simulink model "gm_flyback_pid_vnl"  (R2021b)
settings: Solver=FixedStepDiscrete  StartTime=0.0  StopTime=100e-3  RelTol=1e-3
undefined symbols (not defined in the file or in its folder): DiscIntNeverNeededParam
libraries: simulink x3
Description:
  | Symmetric FIR Filter
  | This example shows how to use HDL Coder(TM) to check, generate,
  | and verify HDL for a fixed-point symmetric FIR filter.
settings Model: Creator=The MathWorks, Inc.  LastModifiedBy=Marco Milanesi
settings SolverCC: AlgebraicLoopSolver=TrustRegion  AutoInsertRateTranBlk=on
settings DataIOCC: LimitDataPoints=on  SaveFormat=Array  SaveOutput=off  SignalLogging=off  SaveTime=off  ReturnWorkspaceOutputs=off  SignalLoggingName=logsOut
settings OptimizationCC: BlockReduction=off  BooleanDataType=off  ConditionallyExecuteInputs=off  DefaultParameterBehavior=Inlined  InheritOutputTypeSmallerThanSingle=on  InlineInvariantSignals=on  ExpressionDepthLimit=2147483647  InitFltsAndDblsToZero=on  LifeSpan=inf  BufferReusableBoundary=off
settings DebuggingCC: AlgebraicLoopMsg=error  SaveWithParameterizedLinksMsg=none  UnderspecifiedInitializationDetection=Classic  MergeDetectMultiDrivingBlocksExec=none  CheckExecutionContextPreStartOutputMsg=on  SignalResolutionControl=TryResolveAllWithWarning  InheritedTsInSrcMsg=none  MultiTaskDSMMsg=warning  MultiTaskCondExecSysMsg=none  SingleTaskRateTransMsg=error  IntegerOverflowMsg=none  ParameterPrecisionLossMsg=none  FcnCallInpInsideContextMsg=warning  BusObjectLabelMismatch=none  StateNameClashWarn=warning  SFUnexpectedBacktrackingDiag=warning  SFNoUnconditionalDefaultTransitionDiag=warning  SFExecutionAtInitializationDiag=none  SFMachineParentedDataDiag=warning  IntegerSaturationMsg=none  ArithmeticOperatorsInVariantConditions=warning
settings HardwareCC: ProdBitPerPointer=32  ProdBitPerSizeT=32  ProdBitPerPtrDiffT=32  ProdLargestAtomicFloat=None  ProdIntDivRoundTo=Undefined  ProdEndianess=Unspecified  ProdWordSize=32  ProdHWDeviceType=ASIC/FPGA  TargetUnknown=on  ProdEqTarget=off
settings ModelReferenceCC: PropagateSignalLabelsOutOfModel=off
settings SFSimCC: SimUseLocalCustomCode=off  CustomCodeUndefinedFunction=UseInterfaceOnly
settings RTWCC: RTWUseLocalCustomCode=off
settings CodeAppCC: StateflowObjectComments=on
settings GRTTargetCC: TargetFcnLib=ansi_tfl_tmw.mat  TargetLangStandard=C89/C90 (ANSI)  CombineOutputUpdateFcns=off  GRTInterface=on
settings ConfigComp: CovMetricSettings=dw  CovSaveCumulativeToWorkspaceVar=on  CovSaveSingleToWorkspaceVar=on  CovExternalEMLEnable=off

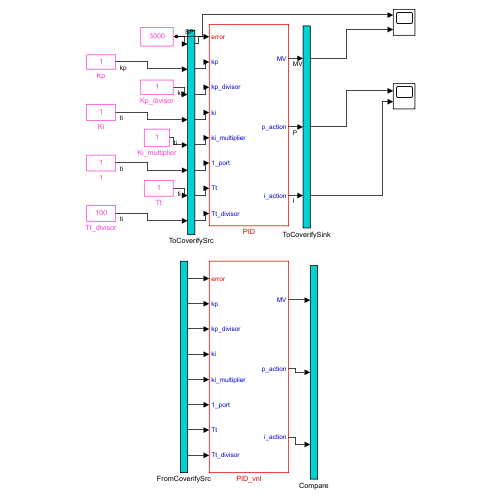
[thumbnail: Simulink's stored preview of the top-level diagram]
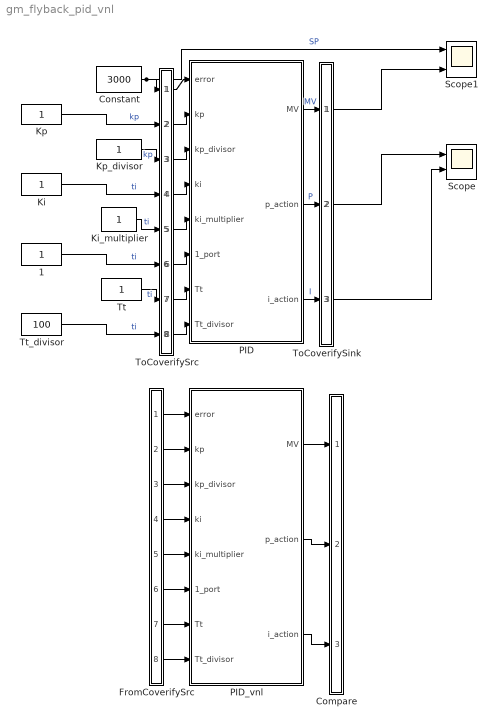
== system gm_flyback_pid_vnl ==
  1 : Constant  OutDataTypeStr=fixdt(1,16,0)
  Compare : Subsystem
      mask Display: disp('')
  Constant : Constant  Value=3000  OutDataTypeStr=fixdt(1,16,0)
  FromCoverifySrc : Subsystem
      mask Display: disp('')
  Ki : Constant  OutDataTypeStr=fixdt(1,16,0)
  Ki_multiplier : Constant  OutDataTypeStr=fixdt(1,16,0)
  Kp : Constant  OutDataTypeStr=fixdt(1,16,0)
  Kp_divisor : Constant  OutDataTypeStr=fixdt(1,16,0)
  PID : Subsystem
  PID_vnl : Subsystem
  Scope : Scope  NumInputPorts=2
  Scope1 : Scope  NumInputPorts=2
  ToCoverifySink : Subsystem
      mask Display: disp('')
  ToCoverifySrc : Subsystem
      mask Display: disp('')
  Tt : Constant  OutDataTypeStr=fixdt(1,16,0)
  Tt_divisor : Constant  Value=100  OutDataTypeStr=fixdt(1,16,0)
  wires:
  Constant/1 -> Scope1/1, ToCoverifySrc/1(in1)  "SP"
  ToCoverifySrc/1(out1) -> PID/1(error)
  ToCoverifySrc/2(out2) -> PID/2(kp)
  ToCoverifySrc/3(out3) -> PID/3(kp_divisor)
  ToCoverifySrc/4(out4) -> PID/4(ki)
  ToCoverifySrc/5(out5) -> PID/5(ki_multiplier)
  ToCoverifySrc/6(out6) -> PID/6(1_port)
  ToCoverifySrc/7(out7) -> PID/7(Tt)
  ToCoverifySrc/8(out8) -> PID/8(Tt_divisor)
  PID/1(MV) -> ToCoverifySink/1(in1)  "MV"
  PID/2(p_action) -> ToCoverifySink/2(in2)  "P"
  PID/3(i_action) -> ToCoverifySink/3(in3)  "I"
  Kp/1 -> ToCoverifySrc/2(in2)  "kp"
  Kp_divisor/1 -> ToCoverifySrc/3(in3)  "kp"
  Ki/1 -> ToCoverifySrc/4(in4)  "ti"
  Ki_multiplier/1 -> ToCoverifySrc/5(in5)  "ti"
  1/1 -> ToCoverifySrc/6(in6)  "ti"
  Tt/1 -> ToCoverifySrc/7(in7)  "ti"
  Tt_divisor/1 -> ToCoverifySrc/8(in8)  "ti"
  ToCoverifySink/1(out1) -> Scope1/2
  ToCoverifySink/2(out2) -> Scope/1
  ToCoverifySink/3(out3) -> Scope/2
  FromCoverifySrc/1(out1) -> PID_vnl/1(error)
  FromCoverifySrc/2(out2) -> PID_vnl/2(kp)
  FromCoverifySrc/3(out3) -> PID_vnl/3(kp_divisor)
  FromCoverifySrc/4(out4) -> PID_vnl/4(ki)
  FromCoverifySrc/5(out5) -> PID_vnl/5(ki_multiplier)
  FromCoverifySrc/6(out6) -> PID_vnl/6(1_port)
  FromCoverifySrc/7(out7) -> PID_vnl/7(Tt)
  FromCoverifySrc/8(out8) -> PID_vnl/8(Tt_divisor)
  PID_vnl/1(MV) -> Compare/1(in1)
  PID_vnl/2(p_action) -> Compare/2(in2)
  PID_vnl/3(i_action) -> Compare/3(in3)

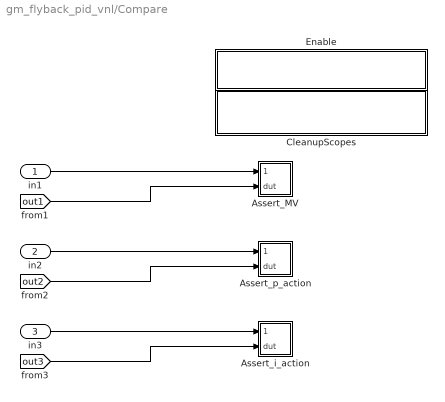
== system gm_flyback_pid_vnl/Compare ==
  in1 : Inport
  in2 : Inport  Port=2
  in3 : Inport  Port=3
  Assert_MV : Subsystem
  Assert_i_action : Subsystem
  Assert_p_action : Subsystem
  CleanupScopes : Subsystem
      settings: OpenFcn=|
      | blkName = gcb; %self block
      | idx = regexp(blkName, '/CleanupScopes$', 'once');
      | blkParent = blkName(1:idx-1);
      | blks=find_system(blkParent, 'LookUnderMasks', 'all','blocktype', 'Scope');
      | for itr = 1:length(blks)
      | 	 hScopeCfg = get_param(blks{itr},'ScopeConfiguration');
      | 	 hScopeCfg.Visible = ~ hScopeCfg.Visible;
      | end
      | drawnow;
      mask Display: fprintf(message('hdlcoder:cosim:vnl_dblclick').getString());
  Enable : Subsystem
      settings: OpenFcn=|
      | blkName = gcb;
      | idx = regexp(blkName, '/Enable$', 'once');
      | blkParent = blkName(1:idx-1);
      | blks=find_system(blkParent, 'LookUnderMasks', 'all','blocktype', 'Assertion');
      | e = get_param(blks{1}, 'Enabled');
      | if strcmp(e, 'on'), f= 'off';, else, f = 'on';, end
      | for ii=1:length(blks), set_param(blks{ii}, 'Enabled', f);, end
      | set_param(gcb, 'MaskDisplay',['fprintf(message(''hdlcoder:cosim:vnl_dblclick_assertions'',','''',upper(e),'''',').getString())']);
      mask Display: fprintf(message('hdlcoder:cosim:vnl_dblclick_assertions','OFF').getString());
  wires:
  in1/1 -> Assert_MV/1(cosim)
  [out1] -> Assert_MV/2(dut)
  in2/1 -> Assert_p_action/1(cosim)
  [out2] -> Assert_p_action/2(dut)
  in3/1 -> Assert_i_action/1(cosim)
  [out3] -> Assert_i_action/2(dut)

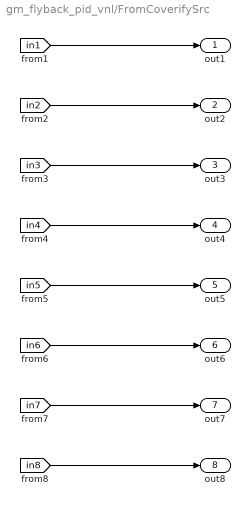
== system gm_flyback_pid_vnl/FromCoverifySrc ==
  out1 : Outport
  out2 : Outport  Port=2
  out3 : Outport  Port=3
  out4 : Outport  Port=4
  out5 : Outport  Port=5
  out6 : Outport  Port=6
  out7 : Outport  Port=7
  out8 : Outport  Port=8
  wires:
  [in1] -> out1/1
  [in2] -> out2/1
  [in3] -> out3/1
  [in4] -> out4/1
  [in5] -> out5/1
  [in6] -> out6/1
  [in7] -> out7/1
  [in8] -> out8/1

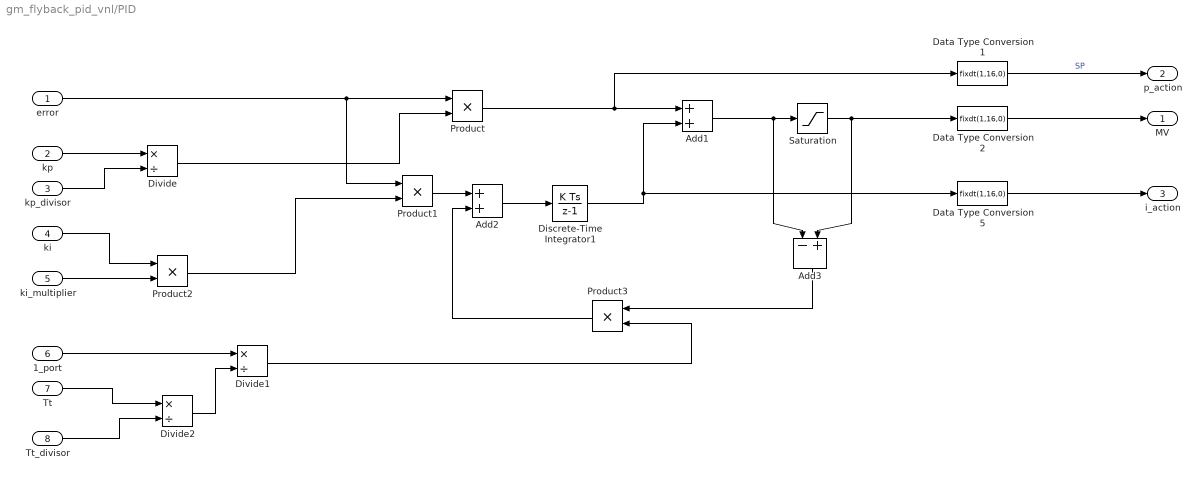
== system gm_flyback_pid_vnl/PID ==
  error : Inport  OutDataTypeStr=fixdt(1,16,0)  SampleTime=80e-9
  kp : Inport  Port=2  OutDataTypeStr=fixdt(1,16,0)  SampleTime=80e-9
  kp_divisor : Inport  Port=3  OutDataTypeStr=fixdt(1,16,0)  SampleTime=80e-9
  ki : Inport  Port=4  OutDataTypeStr=fixdt(1,16,0)  SampleTime=80e-9
  ki_multiplier : Inport  Port=5  OutDataTypeStr=fixdt(1,16,0)  SampleTime=80e-9
  1_port : Inport  Port=6  OutDataTypeStr=fixdt(1,16,0)  SampleTime=80e-9
  Tt : Inport  Port=7  OutDataTypeStr=fixdt(1,16,0)  SampleTime=80e-9
  Tt_divisor : Inport  Port=8  OutDataTypeStr=fixdt(1,16,0)  SampleTime=80e-9
  Add1 : Sum  AccumDataTypeStr=fixdt(1,16,0)  OutDataTypeStr=fixdt(1,16,0)
  Add2 : Sum  AccumDataTypeStr=fixdt(1,16,0)  OutDataTypeStr=fixdt(1,16,0)
  Add3 : Sum  Inputs=-+  AccumDataTypeStr=fixdt(1,16,0)  OutDataTypeStr=fixdt(1,16,0)
  Data Type Conversion1 : DataTypeConversion  OutDataTypeStr=fixdt(1,16,0)
  Data Type Conversion2 : DataTypeConversion  OutDataTypeStr=fixdt(1,16,0)
  Data Type Conversion5 : DataTypeConversion  OutDataTypeStr=fixdt(1,16,0)
  Discrete-Time Integrator1 : DiscreteIntegrator  SampleTime=80e-9  OutDataTypeStr=fixdt(1,16,0)  ICPrevOutput=DiscIntNeverNeededParam  ICPrevScaledInput=DiscIntNeverNeededParam
  Divide : Product  Inputs=*/  OutDataTypeStr=fixdt(1,16,0)  RndMeth=Zero  SaturateOnIntegerOverflow=on
  Divide1 : Product  Inputs=*/  OutDataTypeStr=fixdt(1,16,0)  RndMeth=Zero  SaturateOnIntegerOverflow=on
  Divide2 : Product  Inputs=*/  OutDataTypeStr=fixdt(1,16,0)  RndMeth=Zero  SaturateOnIntegerOverflow=on
  Product{,1..3} (4 alike) : Product  OutDataTypeStr=fixdt(1,16,0)
  Saturation : Saturate  UpperLimit=255  LowerLimit=0  OutDataTypeStr=fixdt(1,16,0)
  MV : Outport  OutDataTypeStr=fixdt(1,16,0)  SampleTime=80e-9  VectorParamsAs1DForOutWhenUnconnected=off
  p_action : Outport  Port=2  OutDataTypeStr=fixdt(1,16,0)  SampleTime=80e-9  VectorParamsAs1DForOutWhenUnconnected=off
  i_action : Outport  Port=3  OutDataTypeStr=fixdt(1,16,0)  SampleTime=80e-9  VectorParamsAs1DForOutWhenUnconnected=off
  wires:
  error/1 -> Product/1, Product1/1
  Product/1 -> Data Type Conversion1/1, Add1/1
  Discrete-Time Integrator1/1 -> Data Type Conversion5/1, Add1/2
  Data Type Conversion1/1 -> p_action/1  "SP"
  Data Type Conversion5/1 -> i_action/1
  Data Type Conversion2/1 -> MV/1
  kp/1 -> Divide/1
  kp_divisor/1 -> Divide/2
  Divide/1 -> Product/2
  ki_multiplier/1 -> Product2/2
  ki/1 -> Product2/1
  Product2/1 -> Product1/2
  Saturation/1 -> Add3/2, Data Type Conversion2/1
  Add1/1 -> Saturation/1, Add3/1
  Product3/1 -> Add2/2
  Add3/1 -> Product3/1
  Product1/1 -> Add2/1
  Add2/1 -> Discrete-Time Integrator1/1
  Divide1/1 -> Product3/2
  Tt_divisor/1 -> Divide2/2
  Tt/1 -> Divide2/1
  1_port/1 -> Divide1/1
  Divide2/1 -> Divide1/2

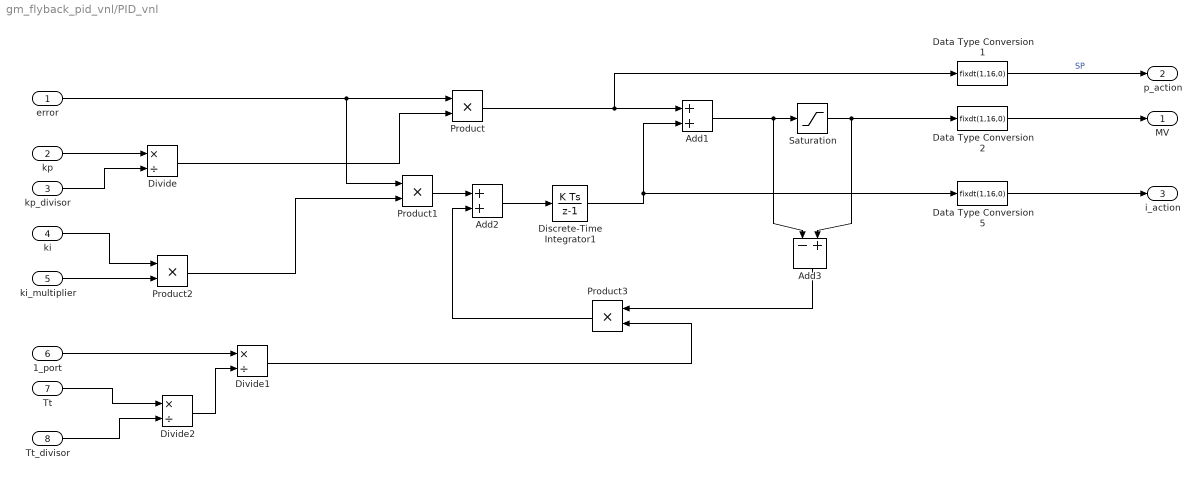
== system gm_flyback_pid_vnl/PID_vnl ==
  error : Inport  OutDataTypeStr=fixdt(1,16,0)  SampleTime=80e-9
  kp : Inport  Port=2  OutDataTypeStr=fixdt(1,16,0)  SampleTime=80e-9
  kp_divisor : Inport  Port=3  OutDataTypeStr=fixdt(1,16,0)  SampleTime=80e-9
  ki : Inport  Port=4  OutDataTypeStr=fixdt(1,16,0)  SampleTime=80e-9
  ki_multiplier : Inport  Port=5  OutDataTypeStr=fixdt(1,16,0)  SampleTime=80e-9
  1_port : Inport  Port=6  OutDataTypeStr=fixdt(1,16,0)  SampleTime=80e-9
  Tt : Inport  Port=7  OutDataTypeStr=fixdt(1,16,0)  SampleTime=80e-9
  Tt_divisor : Inport  Port=8  OutDataTypeStr=fixdt(1,16,0)  SampleTime=80e-9
  Add1 : Sum  AccumDataTypeStr=fixdt(1,16,0)  OutDataTypeStr=fixdt(1,16,0)
  Add2 : Sum  AccumDataTypeStr=fixdt(1,16,0)  OutDataTypeStr=fixdt(1,16,0)
  Add3 : Sum  Inputs=-+  AccumDataTypeStr=fixdt(1,16,0)  OutDataTypeStr=fixdt(1,16,0)
  Data Type Conversion1 : DataTypeConversion  OutDataTypeStr=fixdt(1,16,0)
  Data Type Conversion2 : DataTypeConversion  OutDataTypeStr=fixdt(1,16,0)
  Data Type Conversion5 : DataTypeConversion  OutDataTypeStr=fixdt(1,16,0)
  Discrete-Time Integrator1 : DiscreteIntegrator  SampleTime=80e-9  OutDataTypeStr=fixdt(1,16,0)  ICPrevOutput=DiscIntNeverNeededParam  ICPrevScaledInput=DiscIntNeverNeededParam
  Divide : Product  Inputs=*/  OutDataTypeStr=fixdt(1,16,0)  RndMeth=Zero  SaturateOnIntegerOverflow=on
  Divide1 : Product  Inputs=*/  OutDataTypeStr=fixdt(1,16,0)  RndMeth=Zero  SaturateOnIntegerOverflow=on
  Divide2 : Product  Inputs=*/  OutDataTypeStr=fixdt(1,16,0)  RndMeth=Zero  SaturateOnIntegerOverflow=on
  Product{,1..3} (4 alike) : Product  OutDataTypeStr=fixdt(1,16,0)
  Saturation : Saturate  UpperLimit=255  LowerLimit=0  OutDataTypeStr=fixdt(1,16,0)
  MV : Outport  OutDataTypeStr=fixdt(1,16,0)  SampleTime=80e-9  VectorParamsAs1DForOutWhenUnconnected=off
  p_action : Outport  Port=2  OutDataTypeStr=fixdt(1,16,0)  SampleTime=80e-9  VectorParamsAs1DForOutWhenUnconnected=off
  i_action : Outport  Port=3  OutDataTypeStr=fixdt(1,16,0)  SampleTime=80e-9  VectorParamsAs1DForOutWhenUnconnected=off
  wires:
  Divide2/1 -> Divide1/2
  1_port/1 -> Divide1/1
  Tt/1 -> Divide2/1
  Tt_divisor/1 -> Divide2/2
  Divide1/1 -> Product3/2
  Add2/1 -> Discrete-Time Integrator1/1
  Product1/1 -> Add2/1
  Add3/1 -> Product3/1
  Product3/1 -> Add2/2
  Add1/1 -> Add3/1, Saturation/1
  Saturation/1 -> Data Type Conversion2/1, Add3/2
  Product2/1 -> Product1/2
  ki/1 -> Product2/1
  ki_multiplier/1 -> Product2/2
  Divide/1 -> Product/2
  kp_divisor/1 -> Divide/2
  kp/1 -> Divide/1
  Data Type Conversion2/1 -> MV/1
  Data Type Conversion5/1 -> i_action/1
  Data Type Conversion1/1 -> p_action/1  "SP"
  Discrete-Time Integrator1/1 -> Add1/2, Data Type Conversion5/1
  Product/1 -> Add1/1, Data Type Conversion1/1
  error/1 -> Product1/1, Product/1

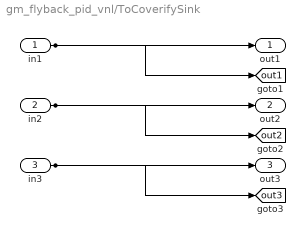
== system gm_flyback_pid_vnl/ToCoverifySink ==
  in1 : Inport
  in2 : Inport  Port=2
  in3 : Inport  Port=3
  out1 : Outport
  out2 : Outport  Port=2
  out3 : Outport  Port=3
  tag scope: out1=global, out2=global, out3=global
  wires:
  in1/1 -> out1/1, [out1]
  in2/1 -> out2/1, [out2]
  in3/1 -> out3/1, [out3]

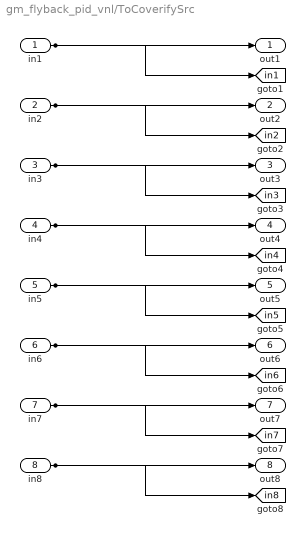
== system gm_flyback_pid_vnl/ToCoverifySrc ==
  in1 : Inport
  in2 : Inport  Port=2
  in3 : Inport  Port=3
  in4 : Inport  Port=4
  in5 : Inport  Port=5
  in6 : Inport  Port=6
  in7 : Inport  Port=7
  in8 : Inport  Port=8
  out1 : Outport
  out2 : Outport  Port=2
  out3 : Outport  Port=3
  out4 : Outport  Port=4
  out5 : Outport  Port=5
  out6 : Outport  Port=6
  out7 : Outport  Port=7
  out8 : Outport  Port=8
  tag scope: in1=global, in2=global, in3=global, in4=global, in5=global, in6=global, in7=global, in8=global
  wires:
  in1/1 -> out1/1, [in1]
  in2/1 -> out2/1, [in2]
  in3/1 -> out3/1, [in3]
  in4/1 -> out4/1, [in4]
  in5/1 -> out5/1, [in5]
  in6/1 -> out6/1, [in6]
  in7/1 -> out7/1, [in7]
  in8/1 -> out8/1, [in8]

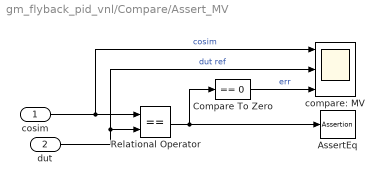
== system gm_flyback_pid_vnl/Compare/Assert_MV ==
  cosim : Inport
  dut : Inport  Port=2
  AssertEq : Assertion  StopWhenAssertionFail=off
  Compare To Zero : simulink/Logic and Bit Operations/Compare To Zero  relop===  OutDataTypeStr=boolean
  Relational Operator : RelationalOperator  Operator===  OutDataTypeStr=boolean  RndMeth=Nearest
  compare: MV : Scope  NumInputPorts=3
  wires:
  Compare To Zero/1 -> compare: MV/3  "err"
  Relational Operator/1 -> Compare To Zero/1, AssertEq/1
  cosim/1 -> compare: MV/1, Relational Operator/1  "cosim"
  dut/1 -> compare: MV/2, Relational Operator/2  "dut ref"

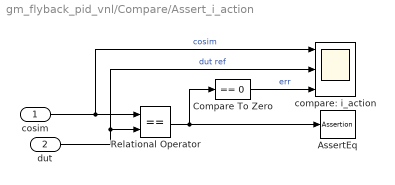
== system gm_flyback_pid_vnl/Compare/Assert_i_action ==
  cosim : Inport
  dut : Inport  Port=2
  AssertEq : Assertion  StopWhenAssertionFail=off
  Compare To Zero : simulink/Logic and Bit Operations/Compare To Zero  relop===  OutDataTypeStr=boolean
  Relational Operator : RelationalOperator  Operator===  OutDataTypeStr=boolean  RndMeth=Nearest
  compare: i_action : Scope  NumInputPorts=3
  wires:
  Compare To Zero/1 -> compare: i_action/3  "err"
  Relational Operator/1 -> Compare To Zero/1, AssertEq/1
  cosim/1 -> compare: i_action/1, Relational Operator/1  "cosim"
  dut/1 -> compare: i_action/2, Relational Operator/2  "dut ref"

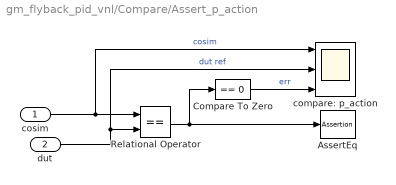
== system gm_flyback_pid_vnl/Compare/Assert_p_action ==
  cosim : Inport
  dut : Inport  Port=2
  AssertEq : Assertion  StopWhenAssertionFail=off
  Compare To Zero : simulink/Logic and Bit Operations/Compare To Zero  relop===  OutDataTypeStr=boolean
  Relational Operator : RelationalOperator  Operator===  OutDataTypeStr=boolean  RndMeth=Nearest
  compare: p_action : Scope  NumInputPorts=3
  wires:
  Compare To Zero/1 -> compare: p_action/3  "err"
  Relational Operator/1 -> Compare To Zero/1, AssertEq/1
  cosim/1 -> compare: p_action/1, Relational Operator/1  "cosim"
  dut/1 -> compare: p_action/2, Relational Operator/2  "dut ref"

== system gm_flyback_pid_vnl/Compare/CleanupScopes ==

== system gm_flyback_pid_vnl/Compare/Enable ==
